simulink model "Solarzelle_Simulink"  (R2022b)
settings: Solver=VariableStepAuto  StartTime=0.0  StopTime=100  RelTol=1e-3
undefined symbols (not defined in the file): param
libraries: simulink x1
settings Model: Creator=chris  LastModifiedBy=milan
settings ModelReferenceCC: EnableRefExpFcnMdlSchedulingChecks=on

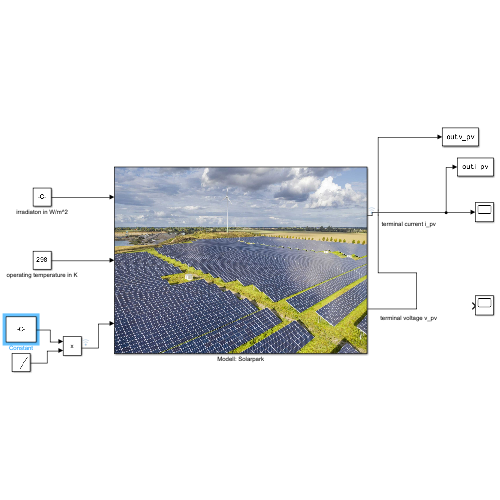
[thumbnail: Simulink's stored preview of the top-level diagram]
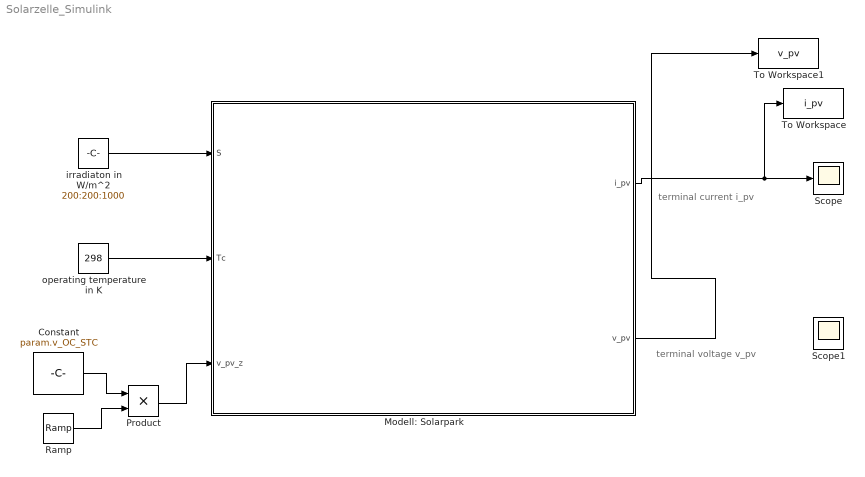
== system Solarzelle_Simulink ==
  note: terminal voltage v_pv
  note: terminal current i_pv
  Constant : Constant  Value=param.v_OC_STC
  Modell: Solarpark : Subsystem
      mask Display: image('$imagefile'); % Use "Edit Image" on toolstrip to change.
  Product : Product
  Ramp : simulink/Sources/Ramp  slope=1/100  start=0  InitialOutput=0
  Scope : Scope
  Scope1 : Scope
  To Workspace : ToWorkspace  VariableName=i_pv  SaveFormat=Timeseries  SampleTime=-1
  To Workspace1 : ToWorkspace  VariableName=v_pv  SaveFormat=Timeseries  SampleTime=-1
  irradiaton in W/m^2 : Constant  Value=200:200:1000
  operating temperature in K : Constant  Value=298
  wires:
  irradiaton in W/m^2/1 -> Modell: Solarpark/1(S)
  Modell: Solarpark/1(i_pv) -> To Workspace/1, Scope/1
  operating temperature in K/1 -> Modell: Solarpark/2(Tc)
  Product/1 -> Modell: Solarpark/3(v_pv_z)
  Constant/1 -> Product/1
  Ramp/1 -> Product/2
  Modell: Solarpark/2(v_pv) -> To Workspace1/1

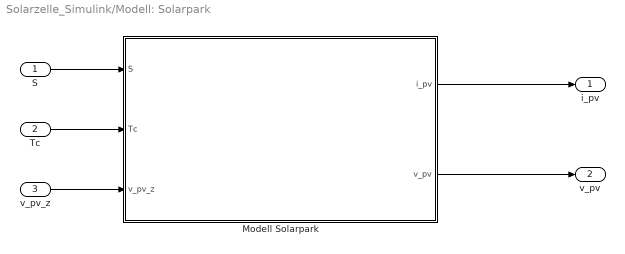
== system Solarzelle_Simulink/Modell: Solarpark ==
  S : Inport
  Tc : Inport  Port=2
  v_pv_z : Inport  Port=3
  Modell Solarpark : MATLAB Function  TreatAsAtomicUnit=on
  i_pv : Outport
  v_pv : Outport  Port=2
  wires:
  Modell Solarpark/1(i_pv) -> i_pv/1
  S/1 -> Modell Solarpark/1(S)
  Tc/1 -> Modell Solarpark/2(Tc)
  v_pv_z/1 -> Modell Solarpark/3(v_pv_z)
  Modell Solarpark/2(v_pv) -> v_pv/1

== matlab function Solarzelle_Simulink/Modell: Solarpark/Modell Solarpark ==
  data: S input; i_pv output; param parameter; Tc input; v_pv_z input; v_pv output
function [i_pv,v_pv]  = fcn(S, param, Tc,v_pv_z) 

% 1. Gleichung: Photodiodenstrom
i_ph = S/param.S_STC * param.iph_SC_STC *(1 + param.alpha_T * (Tc-param.Tc_STC)); 

%Berechnung der Leerlaufspannung für i_s
v_OC = param.v_OC_STC * (1 + param.beta_T * (Tc-param.Tc_STC));

% 2. Gleichung: Irgendwas Strom
i_s = (i_ph - (v_OC/param.Rh))/(exp(v_OC/(param.An * param.vT_STC))-1);

% 3. Gleichung: Bypass-Diodenstrom
i_d = i_s * (exp(v_pv_z/(param.An*param.vT_STC))-1);

% Resultierender Strom aller paralellgeschalteter Solarzellen;
i_pv = param.Np * i_ph - param.Np * i_d - (param.Np/param.Ns) * (v_pv_z/param.Rh);

%Resultierende Spannungswerte aller in reihegeschalteter Solarzellen
v_pv = param.Ns * v_pv_z;

end
